simulink model "sensorsTestHarness"  (R2024a)
settings: configuration reference "standardSILConfiguraitonParams" (kept outside this file)
settings Model: Creator=aeroth  LastModifiedBy=jerem
settings ConfigSetRef: SourceName=standardSILConfiguraitonParams  SourceLocation=Base Workspace

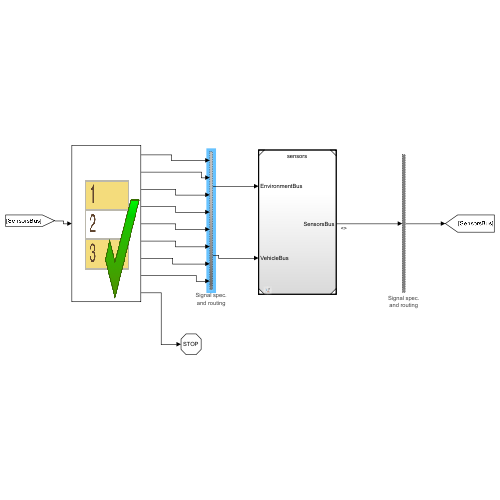
[thumbnail: Simulink's stored preview of the top-level diagram]
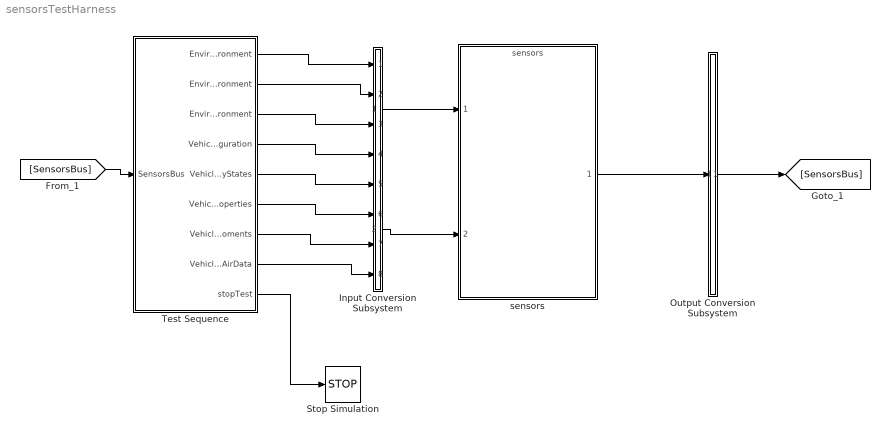
== system sensorsTestHarness ==
  Input Conversion Subsystem : Subsystem  Tag=__SLT_ICS__  Description=|
      | Signal spec.
      | and routing
      settings: AttributesFormatString=%<Description>
  Output Conversion Subsystem : Subsystem  Tag=__SLT_OCS__  Description=|
      | Signal spec.
      | and routing
      mask init:
      | ICDictionary = get_param(bdroot, 'DataDictionary');
      | if isempty(ICDictionary)
      |    ICScope = Simulink.data.BaseWorkspace;
      | else
      |    ICScope = Simulink.data.DataDictionary(ICDictionary);
      | end
      | 
      | IC1 = Simulink.Bus.createMATLABStruct('SensorsBus', [], [1 1], ICScope);
      settings: AttributesFormatString=%<Description>
  Stop Simulation : Stop
  Test Sequence : Test Sequence  TreatAsAtomicUnit=on  SystemSampleTime=0.2
  sensors : ModelReference  ModelNameDialog=sensors  SimulationMode=Normal  ModelReferenceVersion=1.27
  wires:
  Test Sequence/1(EnvironmentBus_EarthEnvironment) -> Input Conversion Subsystem/1(Inport_1)
  Test Sequence/2(EnvironmentBus_AirEnvironment) -> Input Conversion Subsystem/2(Inport_2)
  Test Sequence/3(EnvironmentBus_TerrainEnvironment) -> Input Conversion Subsystem/3(Inport_3)
  Test Sequence/4(VehicleBus_VehicleConfiguration) -> Input Conversion Subsystem/4(Inport_4)
  Test Sequence/5(VehicleBus_BodyStates) -> Input Conversion Subsystem/5(Inport_5)
  Test Sequence/6(VehicleBus_MassProperties) -> Input Conversion Subsystem/6(Inport_6)
  Test Sequence/7(VehicleBus_AircraftForcesMoments) -> Input Conversion Subsystem/7(Inport_7)
  Test Sequence/8(VehicleBus_AirData) -> Input Conversion Subsystem/8(Inport_8)
  [SensorsBus] -> Test Sequence/1(SensorsBus)
  Output Conversion Subsystem/1(Outport_1) -> [SensorsBus]
  Test Sequence/9(stopTest) -> Stop Simulation/1
  sensors/1 -> Output Conversion Subsystem/1(Inport_1)
  Input Conversion Subsystem/1(Outport_1) -> sensors/1
  Input Conversion Subsystem/2(Outport_2) -> sensors/2

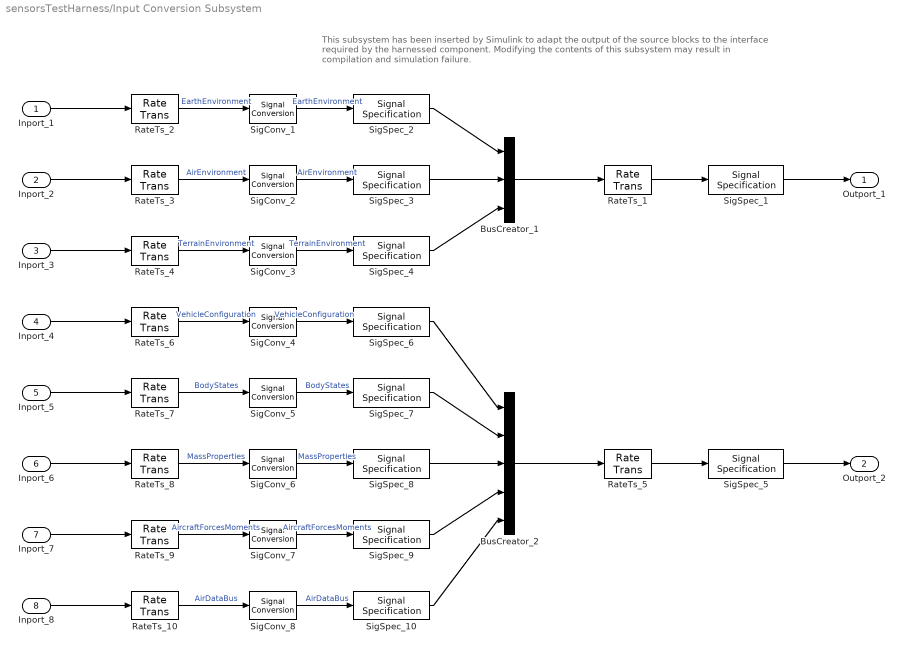
== system sensorsTestHarness/Input Conversion Subsystem ==
  note: This subsystem has been inserted by Simulink to adapt the output of the source blocks to the interface required by the harnessed component.
      |  Modifying the contents of this subsystem may result in compilation and simulation failure.
  Inport_1 : Inport
  Inport_2 : Inport  Port=2
  Inport_3 : Inport  Port=3
  Inport_4 : Inport  Port=4
  Inport_5 : Inport  Port=5
  Inport_6 : Inport  Port=6
  Inport_7 : Inport  Port=7
  Inport_8 : Inport  Port=8
  BusCreator_1 : BusCreator  Inputs=3  OutDataTypeStr=Bus: EnvironmentBus
  BusCreator_2 : BusCreator  Inputs=5  OutDataTypeStr=Bus: VehicleBus
  RateTs_{1..10} (10 alike) : RateTransition  OutPortSampleTime=0.004
  SigConv_{1..8} (8 alike) : SignalConversion  ConversionOutput=Nonvirtual bus  OverrideOpt=off
  SigSpec_1 : SignalSpecification  OutDataTypeStr=Bus: EnvironmentBus  SampleTime=0.004
  SigSpec_10 : SignalSpecification  OutDataTypeStr=Bus: AirDataBus  Dimensions=[1]  BusOutputAsStruct=on
  SigSpec_2 : SignalSpecification  OutDataTypeStr=Bus: EarthEnvironmentBus  Dimensions=[1]  SampleTime=0.004  BusOutputAsStruct=on
  SigSpec_3 : SignalSpecification  OutDataTypeStr=Bus: AirEnvironmentBus  Dimensions=[1]  SampleTime=0.004  BusOutputAsStruct=on
  SigSpec_4 : SignalSpecification  OutDataTypeStr=Bus: TerrainEnvironmentBus  Dimensions=[1]  SampleTime=0.004  BusOutputAsStruct=on
  SigSpec_5 : SignalSpecification  OutDataTypeStr=Bus: VehicleBus  SampleTime=0.004
  SigSpec_6 : SignalSpecification  OutDataTypeStr=Bus: VehicleConfigurationBus  Dimensions=[1]  SampleTime=0.004  BusOutputAsStruct=on
  SigSpec_7 : SignalSpecification  OutDataTypeStr=Bus: BodyStateBus  Dimensions=[1]  SampleTime=0.004  BusOutputAsStruct=on
  SigSpec_8 : SignalSpecification  OutDataTypeStr=Bus: MassPropertiesBus  Dimensions=[1]  SampleTime=0.004  BusOutputAsStruct=on
  SigSpec_9 : SignalSpecification  OutDataTypeStr=Bus: AircraftForcesMomentsBus  Dimensions=[1]  SampleTime=0.004  BusOutputAsStruct=on
  Outport_1 : Outport
  Outport_2 : Outport  Port=2
  wires:
  SigSpec_1/1 -> Outport_1/1
  RateTs_1/1 -> SigSpec_1/1
  BusCreator_1/1 -> RateTs_1/1
  SigSpec_2/1 -> BusCreator_1/1
  SigConv_1/1 -> SigSpec_2/1  "EarthEnvironment"
  RateTs_2/1 -> SigConv_1/1  "EarthEnvironment"
  Inport_1/1 -> RateTs_2/1
  SigSpec_3/1 -> BusCreator_1/2
  SigConv_2/1 -> SigSpec_3/1  "AirEnvironment"
  RateTs_3/1 -> SigConv_2/1  "AirEnvironment"
  Inport_2/1 -> RateTs_3/1
  SigSpec_4/1 -> BusCreator_1/3
  SigConv_3/1 -> SigSpec_4/1  "TerrainEnvironment"
  RateTs_4/1 -> SigConv_3/1  "TerrainEnvironment"
  Inport_3/1 -> RateTs_4/1
  SigSpec_5/1 -> Outport_2/1
  RateTs_5/1 -> SigSpec_5/1
  BusCreator_2/1 -> RateTs_5/1
  SigSpec_6/1 -> BusCreator_2/1
  SigConv_4/1 -> SigSpec_6/1  "VehicleConfiguration"
  RateTs_6/1 -> SigConv_4/1  "VehicleConfiguration"
  Inport_4/1 -> RateTs_6/1
  SigSpec_7/1 -> BusCreator_2/2
  SigConv_5/1 -> SigSpec_7/1  "BodyStates"
  RateTs_7/1 -> SigConv_5/1  "BodyStates"
  Inport_5/1 -> RateTs_7/1
  SigSpec_8/1 -> BusCreator_2/3
  SigConv_6/1 -> SigSpec_8/1  "MassProperties"
  RateTs_8/1 -> SigConv_6/1  "MassProperties"
  Inport_6/1 -> RateTs_8/1
  SigSpec_9/1 -> BusCreator_2/4
  SigConv_7/1 -> SigSpec_9/1  "AircraftForcesMoments"
  RateTs_9/1 -> SigConv_7/1  "AircraftForcesMoments"
  Inport_7/1 -> RateTs_9/1
  SigSpec_10/1 -> BusCreator_2/5
  SigConv_8/1 -> SigSpec_10/1  "AirDataBus"
  RateTs_10/1 -> SigConv_8/1  "AirDataBus"
  Inport_8/1 -> RateTs_10/1

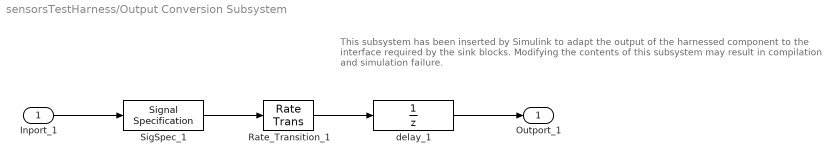
== system sensorsTestHarness/Output Conversion Subsystem ==
  note: This subsystem has been inserted by Simulink to adapt the output of the harnessed component to the interface required by the sink blocks.
      |  Modifying the contents of this subsystem may result in compilation and simulation failure.
  Inport_1 : Inport
  Rate_Transition_1 : RateTransition  OutPortSampleTimeOpt=Inherit
  SigSpec_1 : SignalSpecification  OutDataTypeStr=Bus: SensorsBus  Dimensions=[1]  SampleTime=0.004  BusOutputAsStruct=on
  delay_1 : UnitDelay  InitialCondition=IC1  SampleTime=-1
  Outport_1 : Outport
  wires:
  Inport_1/1 -> SigSpec_1/1
  SigSpec_1/1 -> Rate_Transition_1/1
  Rate_Transition_1/1 -> delay_1/1
  delay_1/1 -> Outport_1/1

== stateflow chart sensorsTestHarness/Test Sequence ==
  state Scenario_1
    state Initialize
      %% Initialize data outputs.
      stopTest = false;
      EnvironmentBus_EarthEnvironment.gravityScalar_mps2 = 0;
      EnvironmentBus_AirEnvironment.airTemperature_K = 0;
      EnvironmentBus_AirEnvironment.airPressure_Pa = 0;
      EnvironmentBus_AirEnvironment.airDensity_kgpm3 = 0;
      EnvironmentBus_AirEnvironment.windSpeedInNED_mps = zeros(3,1);
      EnvironmentBus_AirEnvironment.speedOfSound_mps = 0;
      EnvironmentBus_TerrainEnvironment.terrainHeightInNED_m = 0;
      VehicleBus_VehicleConfiguration.isVehicleAirborne = false;
      VehicleBus_BodyStates.aircraftVelInNED_mps = zeros(3,1);
      VehicleBus_BodyStates.aircraftPosInNED_m = zeros(3,1);
      VehicleBus_BodyStates.aircraftEulerAngles_rad = zeros(3,1);
      VehicleBus_BodyStates.aircraftVelInBody_mps = zeros(3,1);
      VehicleBus_BodyStates.aircraftAngVelInBody_radps = zeros(3,1);
      VehicleBus_BodyStates.aircraftAngAccelInBody_radps2 = zeros(3,1);
      VehicleBus_BodyStates.aircraftAccelInBody_mps2 = zeros(3,1);
      VehicleBus_BodyStates.DCM_be = zeros(3,3);
      VehicleBus_MassProperties.aircraftMass_kg = 0;
      VehicleBus_MassProperties.aircraftCg_m = zeros(3,1);
      VehicleBus_MassProperties.aircraftInertiaInBody_kgm2 = zeros(3,3);
      VehicleBus_AircraftForcesMoments.forcesInBody_N = zeros(3,1);
      VehicleBus_AircraftForcesMoments.momentsInBody_Nm = zeros(3,1);
      VehicleBus_AircraftForcesMoments.aeroForcesMoments.forcesInBody_N = zeros(3,1);
      VehicleBus_AircraftForcesMoments.aeroForcesMoments.momentsInBody_Nm = zeros(3,1);
      VehicleBus_AircraftForcesMoments.engineForcesMoments.forcesInBody_N = zeros(3,1);
      VehicleBus_AircraftForcesMoments.engineForcesMoments.momentsInBody_Nm = zeros(3,1);
      VehicleBus_AircraftForcesMoments.groundForcesMoments.forcesInBody_N = zeros(3,1);
      VehicleBus_AircraftForcesMoments.groundForcesMoments.momentsInBody_Nm = zeros(3,1);
      VehicleBus_AirData.airspeedInBody_mps = zeros(3,1);
      VehicleBus_AirData.alpha_rad = 0;
      VehicleBus_AirData.beta_rad = 0;
    state EndTest
      stopTest = true;
    (default) -> Initialize
    Initialize -> EndTest : [
        | true
        | ]
  (default) -> Scenario_1 : {assert(Active_Scenario_Index == 1,'The value of Scenario Parameter ''Active_Scenario_Index'' is not valid. Use the index of the scenario to specify it.')}
  data: SensorsBus input Bus: SensorsBus size=[1]; EnvironmentBus_EarthEnvironment output Bus: EarthEnvironmentBus size=[1]; EnvironmentBus_AirEnvironment output Bus: AirEnvironmentBus size=[1]; EnvironmentBus_TerrainEnvironment output Bus: TerrainEnvironmentBus size=[1]; VehicleBus_VehicleConfiguration output Bus: VehicleConfigurationBus size=[1]; VehicleBus_BodyStates output Bus: BodyStateBus size=[1]; VehicleBus_MassProperties output Bus: MassPropertiesBus size=[1]; VehicleBus_AircraftForcesMoments output Bus: AircraftForcesMomentsBus size=[1]; VehicleBus_AirData output Bus: AirDataBus size=[1]; Active_Scenario_Index parameter =1; stopTest output
